simulink model "hw2_q4_2"  (R2018b)
settings: Solver=VariableStepAuto  StartTime=-5  StopTime=100  RelTol=1e-3
settings Model: Creator=Sazgar Shargh  LastModifiedBy=Sazgar Shargh

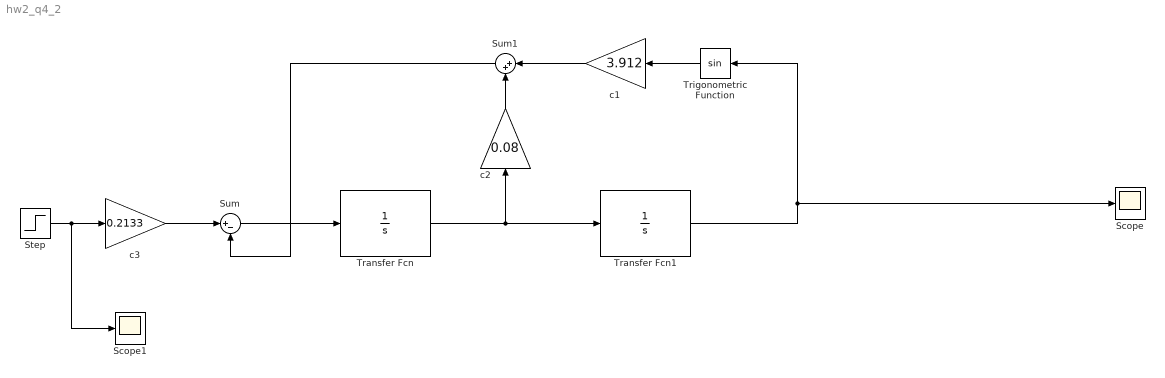
== system hw2_q4_2 ==
  Scope : Scope
  Scope1 : Scope
  Step : Step  Time=0.00001  After=200  SampleTime=0
  Sum : Sum  Inputs=|+-
  Sum1 : Sum  Inputs=|++
  Transfer Fcn : TransferFcn  Denominator=[1 0]
  Transfer Fcn1 : TransferFcn  Denominator=[1 0]
  Trigonometric Function : Trigonometry
  c1 : Gain  Gain=3.912
  c2 : Gain  Gain=0.08
  c3 : Gain  Gain=0.2133
  wires:
  c3/1 -> Sum/1
  Step/1 -> Scope1/1, c3/1
  Sum/1 -> Transfer Fcn/1
  Transfer Fcn/1 -> c2/1, Transfer Fcn1/1
  c2/1 -> Sum1/2
  c1/1 -> Sum1/1
  Trigonometric Function/1 -> c1/1
  Sum1/1 -> Sum/2
  Transfer Fcn1/1 -> Scope/1, Trigonometric Function/1
